simulink library "Bit_Multiplexers_Lib"  (R2023a)
settings: Solver=ode45  StartTime=0.0  StopTime=10.0  RelTol=1e-3  EnableMultiTasking=on
settings Model: Creator=uzivatel  LastModifiedBy=Jozko Mrkvicka
settings SolverCC: AlgebraicLoopSolver=TrustRegion
settings DataIOCC: LimitDataPoints=on  SaveFormat=Array  ReturnWorkspaceOutputs=off
settings OptimizationCC: LifeSpan=inf
settings DebuggingCC: UnderspecifiedInitializationDetection=Classic  MergeDetectMultiDrivingBlocksExec=none  SolverPrmCheckMsg=warning  UnconnectedInputMsg=warning  UnconnectedOutputMsg=warning  UnconnectedLineMsg=warning  StateNameClashWarn=warning  SFUnexpectedBacktrackingDiag=warning  SFNoUnconditionalDefaultTransitionDiag=warning  ArithmeticOperatorsInVariantConditions=warning
settings HardwareCC: ProdBitPerPointer=32  ProdBitPerSizeT=32  ProdBitPerPtrDiffT=32  ProdLargestAtomicFloat=None  ProdIntDivRoundTo=Undefined  ProdEndianess=Unspecified  ProdWordSize=32  ProdHWDeviceType=32-bit Generic
settings ModelReferenceCC: EnableRefExpFcnMdlSchedulingChecks=on  PropagateSignalLabelsOutOfModel=off
settings SFSimCC: SimUseLocalCustomCode=off  CustomCodeUndefinedFunction=UseInterfaceOnly
settings RTWCC: RTWUseLocalCustomCode=off
settings CodeAppCC: StateflowObjectComments=on
settings GRTTargetCC: TargetLangStandard=C89/C90 (ANSI)
settings ConfigComp: CovMetricSettings=dw  CovSaveCumulativeToWorkspaceVar=on  CovSaveSingleToWorkspaceVar=on  CovExternalEMLEnable=off

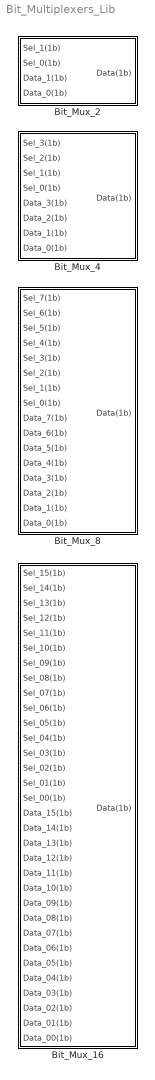
== system Bit_Multiplexers_Lib ==
  Bit_Mux_16 : Subsystem
  Bit_Mux_2 : Subsystem
  Bit_Mux_4 : Subsystem
  Bit_Mux_8 : Subsystem

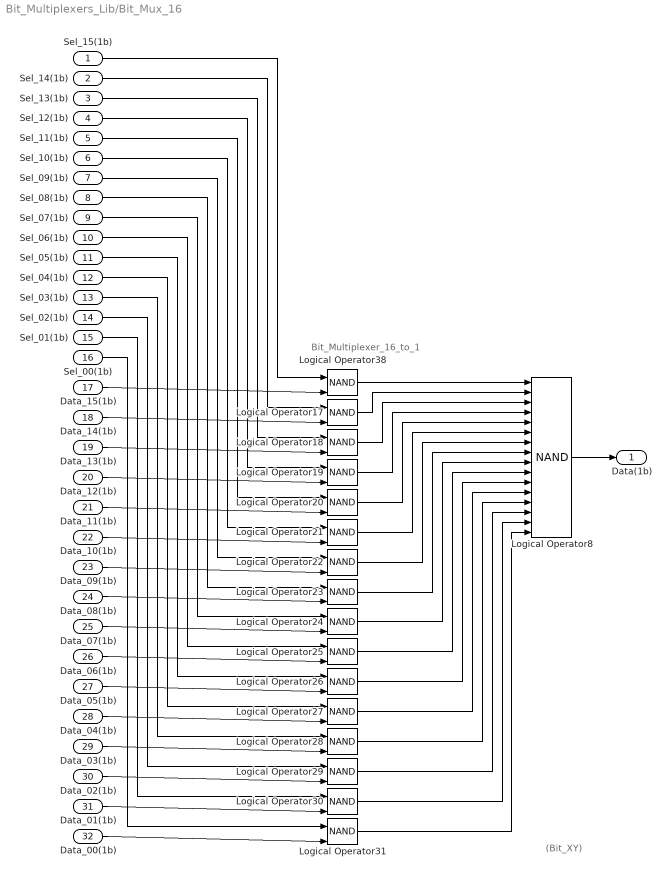
== system Bit_Multiplexers_Lib/Bit_Mux_16 ==
  note: Bit_Multiplexer_16_to_1
  note: (Bit_XY)
  Sel_15(1b) : Inport
  Sel_14(1b) : Inport  Port=2
  Sel_13(1b) : Inport  Port=3
  Sel_12(1b) : Inport  Port=4
  Sel_11(1b) : Inport  Port=5
  Sel_10(1b) : Inport  Port=6
  Sel_09(1b) : Inport  Port=7
  Sel_08(1b) : Inport  Port=8
  Sel_07(1b) : Inport  Port=9
  Sel_06(1b) : Inport  Port=10
  Sel_05(1b) : Inport  Port=11
  Sel_04(1b) : Inport  Port=12
  Sel_03(1b) : Inport  Port=13
  Sel_02(1b) : Inport  Port=14
  Sel_01(1b) : Inport  Port=15
  Sel_00(1b) : Inport  Port=16
  Data_15(1b) : Inport  Port=17
  Data_14(1b) : Inport  Port=18
  Data_13(1b) : Inport  Port=19
  Data_12(1b) : Inport  Port=20
  Data_11(1b) : Inport  Port=21
  Data_10(1b) : Inport  Port=22
  Data_09(1b) : Inport  Port=23
  Data_08(1b) : Inport  Port=24
  Data_07(1b) : Inport  Port=25
  Data_06(1b) : Inport  Port=26
  Data_05(1b) : Inport  Port=27
  Data_04(1b) : Inport  Port=28
  Data_03(1b) : Inport  Port=29
  Data_02(1b) : Inport  Port=30
  Data_01(1b) : Inport  Port=31
  Data_00(1b) : Inport  Port=32
  Logical Operator{17..31,38} (16 alike) : Logic  Operator=NAND  IconShape=distinctive  AllPortsSameDT=off  OutDataTypeStr=boolean
  Logical Operator8 : Logic  Operator=NAND  Inputs=16  IconShape=distinctive  OutDataTypeStr=boolean
  Data(1b) : Outport
  wires:
  Data_03(1b)/1 -> Logical Operator28/2
  Logical Operator28/1 -> Logical Operator8/13
  Logical Operator8/1 -> Data(1b)/1
  Data_09(1b)/1 -> Logical Operator22/2
  Logical Operator20/1 -> Logical Operator8/5
  Data_14(1b)/1 -> Logical Operator17/2
  Logical Operator38/1 -> Logical Operator8/1
  Data_04(1b)/1 -> Logical Operator27/2
  Logical Operator19/1 -> Logical Operator8/4
  Data_08(1b)/1 -> Logical Operator23/2
  Logical Operator25/1 -> Logical Operator8/10
  Logical Operator27/1 -> Logical Operator8/12
  Logical Operator18/1 -> Logical Operator8/3
  Data_00(1b)/1 -> Logical Operator31/2
  Logical Operator17/1 -> Logical Operator8/2
  Data_05(1b)/1 -> Logical Operator26/2
  Logical Operator24/1 -> Logical Operator8/9
  Data_13(1b)/1 -> Logical Operator18/2
  Logical Operator30/1 -> Logical Operator8/15
  Logical Operator21/1 -> Logical Operator8/6
  Data_01(1b)/1 -> Logical Operator30/2
  Data_07(1b)/1 -> Logical Operator24/2
  Data_15(1b)/1 -> Logical Operator38/2
  Logical Operator31/1 -> Logical Operator8/16
  Data_06(1b)/1 -> Logical Operator25/2
  Data_11(1b)/1 -> Logical Operator20/2
  Logical Operator26/1 -> Logical Operator8/11
  Data_02(1b)/1 -> Logical Operator29/2
  Logical Operator22/1 -> Logical Operator8/7
  Logical Operator29/1 -> Logical Operator8/14
  Logical Operator23/1 -> Logical Operator8/8
  Data_10(1b)/1 -> Logical Operator21/2
  Data_12(1b)/1 -> Logical Operator19/2
  Sel_06(1b)/1 -> Logical Operator25/1
  Sel_03(1b)/1 -> Logical Operator28/1
  Sel_10(1b)/1 -> Logical Operator21/1
  Sel_02(1b)/1 -> Logical Operator29/1
  Sel_07(1b)/1 -> Logical Operator24/1
  Sel_05(1b)/1 -> Logical Operator26/1
  Sel_04(1b)/1 -> Logical Operator27/1
  Sel_09(1b)/1 -> Logical Operator22/1
  Sel_14(1b)/1 -> Logical Operator17/1
  Sel_13(1b)/1 -> Logical Operator18/1
  Sel_11(1b)/1 -> Logical Operator20/1
  Sel_01(1b)/1 -> Logical Operator30/1
  Sel_15(1b)/1 -> Logical Operator38/1
  Sel_00(1b)/1 -> Logical Operator31/1
  Sel_08(1b)/1 -> Logical Operator23/1
  Sel_12(1b)/1 -> Logical Operator19/1

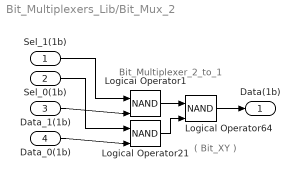
== system Bit_Multiplexers_Lib/Bit_Mux_2 ==
  note: Bit_Multiplexer_2_to_1
  note: ( Bit_XY )
  Sel_1(1b) : Inport
  Sel_0(1b) : Inport  Port=2
  Data_1(1b) : Inport  Port=3
  Data_0(1b) : Inport  Port=4
  Logical Operator1 : Logic  Operator=NAND  IconShape=distinctive  AllPortsSameDT=off  OutDataTypeStr=boolean
  Logical Operator21 : Logic  Operator=NAND  IconShape=distinctive  AllPortsSameDT=off  OutDataTypeStr=boolean
  Logical Operator64 : Logic  Operator=NAND  IconShape=distinctive  OutDataTypeStr=boolean
  Data(1b) : Outport
  wires:
  Data_1(1b)/1 -> Logical Operator1/2
  Sel_0(1b)/1 -> Logical Operator21/1
  Data_0(1b)/1 -> Logical Operator21/2
  Sel_1(1b)/1 -> Logical Operator1/1
  Logical Operator64/1 -> Data(1b)/1
  Logical Operator21/1 -> Logical Operator64/2
  Logical Operator1/1 -> Logical Operator64/1

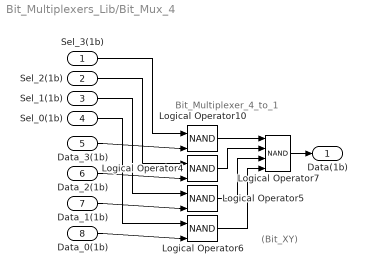
== system Bit_Multiplexers_Lib/Bit_Mux_4 ==
  note: Bit_Multiplexer_4_to_1
  note: (Bit_XY)
  Sel_3(1b) : Inport
  Sel_2(1b) : Inport  Port=2
  Sel_1(1b) : Inport  Port=3
  Sel_0(1b) : Inport  Port=4
  Data_3(1b) : Inport  Port=5
  Data_2(1b) : Inport  Port=6
  Data_1(1b) : Inport  Port=7
  Data_0(1b) : Inport  Port=8
  Logical Operator{4..6,10} (4 alike) : Logic  Operator=NAND  IconShape=distinctive  AllPortsSameDT=off  OutDataTypeStr=boolean
  Logical Operator7 : Logic  Operator=NAND  Inputs=4  IconShape=distinctive  OutDataTypeStr=boolean
  Data(1b) : Outport
  wires:
  Sel_2(1b)/1 -> Logical Operator4/1
  Data_2(1b)/1 -> Logical Operator4/2
  Sel_1(1b)/1 -> Logical Operator5/1
  Sel_3(1b)/1 -> Logical Operator10/1
  Data_0(1b)/1 -> Logical Operator6/2
  Data_3(1b)/1 -> Logical Operator10/2
  Sel_0(1b)/1 -> Logical Operator6/1
  Data_1(1b)/1 -> Logical Operator5/2
  Logical Operator10/1 -> Logical Operator7/1
  Logical Operator5/1 -> Logical Operator7/3
  Logical Operator7/1 -> Data(1b)/1
  Logical Operator4/1 -> Logical Operator7/2
  Logical Operator6/1 -> Logical Operator7/4

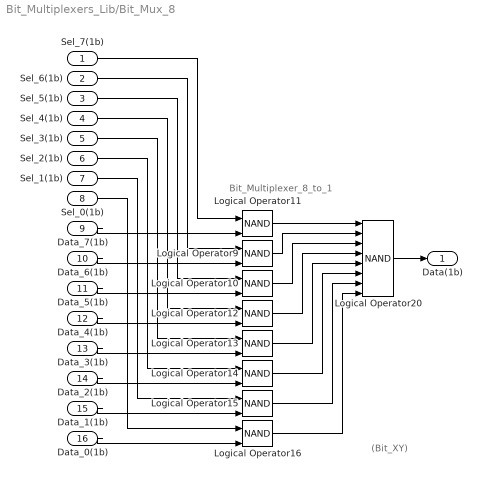
== system Bit_Multiplexers_Lib/Bit_Mux_8 ==
  note: (Bit_XY)
  note: Bit_Multiplexer_8_to_1
  Sel_7(1b) : Inport
  Sel_6(1b) : Inport  Port=2
  Sel_5(1b) : Inport  Port=3
  Sel_4(1b) : Inport  Port=4
  Sel_3(1b) : Inport  Port=5
  Sel_2(1b) : Inport  Port=6
  Sel_1(1b) : Inport  Port=7
  Sel_0(1b) : Inport  Port=8
  Data_7(1b) : Inport  Port=9
  Data_6(1b) : Inport  Port=10
  Data_5(1b) : Inport  Port=11
  Data_4(1b) : Inport  Port=12
  Data_3(1b) : Inport  Port=13
  Data_2(1b) : Inport  Port=14
  Data_1(1b) : Inport  Port=15
  Data_0(1b) : Inport  Port=16
  Logical Operator{9..16} (8 alike) : Logic  Operator=NAND  IconShape=distinctive  AllPortsSameDT=off  OutDataTypeStr=boolean
  Logical Operator20 : Logic  Operator=NAND  Inputs=8  IconShape=distinctive  OutDataTypeStr=boolean
  Data(1b) : Outport
  wires:
  Data_3(1b)/1 -> Logical Operator13/2
  Data_4(1b)/1 -> Logical Operator12/2
  Logical Operator11/1 -> Logical Operator20/1
  Logical Operator10/1 -> Logical Operator20/3
  Logical Operator15/1 -> Logical Operator20/7
  Logical Operator9/1 -> Logical Operator20/2
  Logical Operator16/1 -> Logical Operator20/8
  Data_5(1b)/1 -> Logical Operator10/2
  Logical Operator20/1 -> Data(1b)/1
  Data_6(1b)/1 -> Logical Operator9/2
  Logical Operator12/1 -> Logical Operator20/4
  Data_7(1b)/1 -> Logical Operator11/2
  Logical Operator13/1 -> Logical Operator20/5
  Data_2(1b)/1 -> Logical Operator14/2
  Logical Operator14/1 -> Logical Operator20/6
  Data_0(1b)/1 -> Logical Operator16/2
  Data_1(1b)/1 -> Logical Operator15/2
  Sel_0(1b)/1 -> Logical Operator16/1
  Sel_3(1b)/1 -> Logical Operator13/1
  Sel_2(1b)/1 -> Logical Operator14/1
  Sel_1(1b)/1 -> Logical Operator15/1
  Sel_4(1b)/1 -> Logical Operator12/1
  Sel_6(1b)/1 -> Logical Operator9/1
  Sel_7(1b)/1 -> Logical Operator11/1
  Sel_5(1b)/1 -> Logical Operator10/1
